simulink model "qss_example_electric"  (Simulink 9.2)
settings: Solver=VariableStepDiscrete  StartTime=0.0  StopTime=1923  RelTol=1e-3  EnableMultiTasking=on
undefined symbols (not defined in the file or in its folder): g, h, P_aux, r_wheel, rho, speed_m_s, trans_eff
libraries: qss_tb_library_aalto x2
settings Model: Creator=Antti  LastModifiedBy=Jesse
settings DataIOCC: LimitDataPoints=off  SaveOutput=off  SaveTime=off
settings OptimizationCC: BooleanDataType=off  ExpressionDepthLimit=2147483647  InitFltsAndDblsToZero=on
settings DebuggingCC: SaveWithParameterizedLinksMsg=none  SignalResolutionControl=TryResolveAllWithWarning  SolverPrmCheckMsg=warning  MultiTaskDSMMsg=warning  MultiTaskCondExecSysMsg=none
settings GRTTargetCC: TargetFcnLib=ansi_tfl_tmw.mat
settings ConfigComp: CovSFcnEnable=off

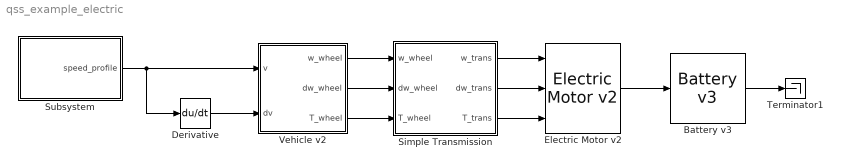
== system qss_example_electric ==
  Battery v3 : qss_tb_library_aalto/Energy Buffer/Battery v3  Tag=battery  init_soc_BT=battery_init_soc  cell_series_BT=192  cell_parallel_BT=25  init_file_BT=battery_file_name
  Derivative : Derivative
  Electric Motor v2 : qss_tb_library_aalto/Energy Converter/Electric Motor v2  scale_EM=3.5  theta_EM=0.5  P_aux=P_aux*1000  over_factor=1.25
  Simple Transmission : Subsystem  Tag=simple transmission  AncestorBlock=qss_tb_library_aalto/Gear System/Simple Transmission  mask(Simple Transmission){gear_ratio=3.5, e_GT=0.98, P_GT0=300, w_wheel_min=1}
      mask prompts: gear_ratio "Gear ratio [-]"; e_GT "Efficiency [-]"; P_GT0 "Idling losses (friction) [W]"; w_wheel_min "Minimum wheel speed beyond which losses are generated [rad/s]"
      mask help:
      | This block simulates a transmission with a fixed gear ratio.
      |
      | Input:
      | =====
      | 	w_wheel	Speed of the wheel [rad/s]
      | 	dw_wheel	Acceleration of the wheel [rad/s^2]
      | 	T_wheel	Torque on the wheel [Nm]
      |
      | Output:
      | ======
      | 	w_trans		Speed of the fly wheel [rad/s]
      | 	dw_trans	Acceleration of the fly wheel [rad/s^2]
      | 	T_trans		Torque on the fly wheel [Nm]
      mask init:
      | init_transmission;
  Subsystem : Subsystem
  Terminator1 : Terminator
  Vehicle v2 : Subsystem  Tag=vehicle  AncestorBlock=qss_tb_library_aalto/Vehicle/Vehicle v2  mask(Vehicle){m_f=1200, mt2m_f=5, A_f=2.0, d_wheel=0.6, cw=0.33, mu=0.01}
      mask prompts: m_f "Total mass of the vehicle [kg]"; mt2m_f "Rotating mass [%]"; A_f "Vehicle cross section [m^2]"; d_wheel "Wheel diameter [m]"; cw "Drag coefficient [-]"; mu "Rolling friction coefficient [-]"
      mask help:
      | This block computes the power required from the vehicle.
      |
      | Input:
      | =====
      | 	v		Speed [m/s]
      | 	dv		Acceleration [m/s^2]
      |
      | Output:
      | ======
      | 	w_wheel	Speed of the wheel [rad/s]
      | 	dw_wheel	Acceleration of the wheel [rad/s^2]
      | 	T_wheel	Torque on the wheel [Nm]
      mask init:
      | init_vehicle_default_v2;
  wires:
  Subsystem/1(speed_profile) -> Vehicle v2/1(v), Derivative/1
  Derivative/1 -> Vehicle v2/2(dv)
  Vehicle v2/1(w_wheel) -> Simple Transmission/1(w_wheel)
  Vehicle v2/2(dw_wheel) -> Simple Transmission/2(dw_wheel)
  Vehicle v2/3(T_wheel) -> Simple Transmission/3(T_wheel)
  Simple Transmission/1(w_trans) -> Electric Motor v2/1
  Simple Transmission/2(dw_trans) -> Electric Motor v2/2
  Simple Transmission/3(T_trans) -> Electric Motor v2/3
  Electric Motor v2/1 -> Battery v3/1
  Battery v3/1 -> Terminator1/1

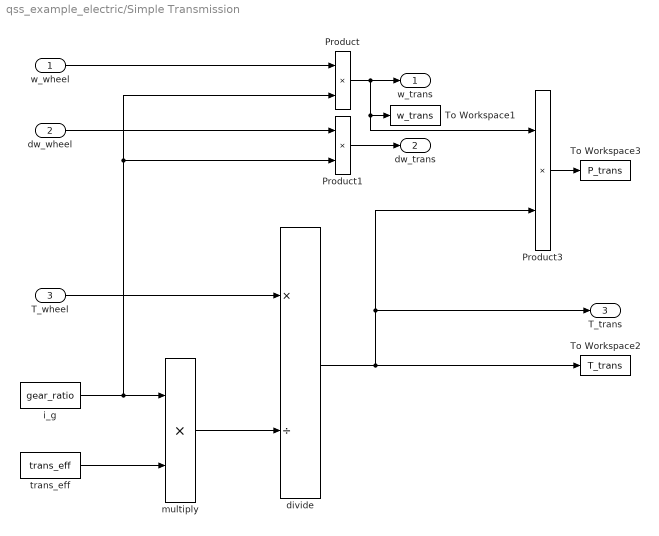
== system qss_example_electric/Simple Transmission ==
  w_wheel : Inport
  dw_wheel : Inport  Port=2
  T_wheel : Inport  Port=3
  Product : Product  SaturateOnIntegerOverflow=on  RndMeth=Zero  InputSameDT=on  OutDataTypeStr=Inherit: Same as first input
  Product1 : Product  SaturateOnIntegerOverflow=on  RndMeth=Zero  InputSameDT=on  OutDataTypeStr=Inherit: Same as first input
  Product3 : Product  SaturateOnIntegerOverflow=on  RndMeth=Zero  InputSameDT=on  OutDataTypeStr=Inherit: Same as first input
  To Workspace1 : ToWorkspace  VariableName=w_trans  SampleTime=-1
  To Workspace2 : ToWorkspace  VariableName=T_trans  SampleTime=-1
  To Workspace3 : ToWorkspace  VariableName=P_trans  SampleTime=-1
  divide : Product  Inputs=*/
  i_g : Constant  Value=gear_ratio
  multiply : Product  Inputs=**
  trans_eff : Constant  Value=trans_eff
  w_trans : Outport  InitialOutput=0
  dw_trans : Outport  Port=2  InitialOutput=0
  T_trans : Outport  Port=3  InitialOutput=0
  wires:
  Product3/1 -> To Workspace3/1
  w_wheel/1 -> Product/1
  dw_wheel/1 -> Product1/1
  Product/1 -> Product3/1, To Workspace1/1, w_trans/1
  Product1/1 -> dw_trans/1
  divide/1 -> Product3/2, T_trans/1, To Workspace2/1
  multiply/1 -> divide/2
  i_g/1 -> Product/2, Product1/2, multiply/1
  trans_eff/1 -> multiply/2
  T_wheel/1 -> divide/1

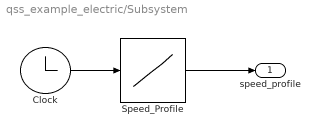
== system qss_example_electric/Subsystem ==
  Clock : Clock
  Speed_Profile : Lookup_n-D  NumberOfTableDimensions=1  BreakpointsSpecification=Even spacing  BreakpointsForDimension1=[0:1923]  Table=speed_m_s  InternalRulePriority=Speed  RndMeth=Simplest  InputSameDT=on
  speed_profile : Outport
  wires:
  Speed_Profile/1 -> speed_profile/1
  Clock/1 -> Speed_Profile/1

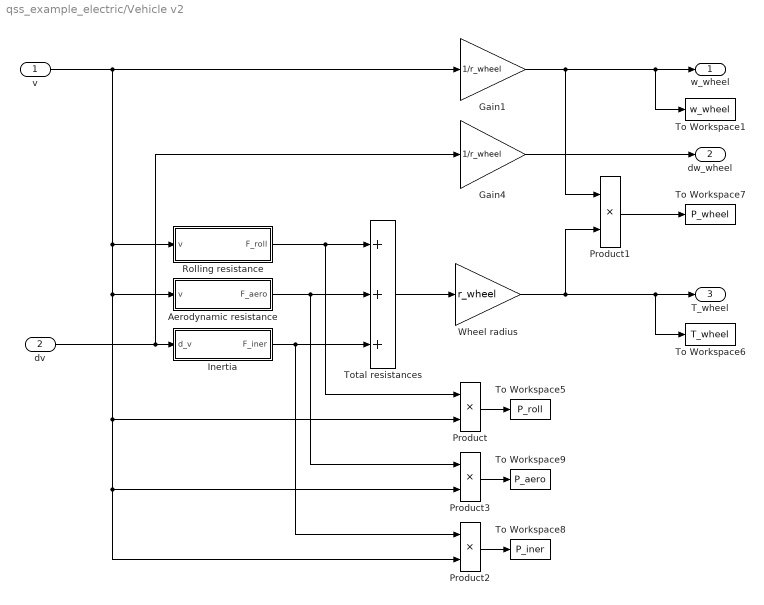
== system qss_example_electric/Vehicle v2 ==
  v : Inport
  dv : Inport  Port=2
  Aerodynamic resistance : Subsystem
  Gain1 : Gain  Gain=1/r_wheel  SaturateOnIntegerOverflow=on  OutDataTypeStr=Inherit: Same as input  ParamDataTypeStr=Inherit: Same as input
  Gain4 : Gain  Gain=1/r_wheel  SaturateOnIntegerOverflow=on  OutDataTypeStr=Inherit: Same as input  ParamDataTypeStr=Inherit: Same as input
  Inertia : Subsystem
  Product{,1..3} (4 alike) : Product  SaturateOnIntegerOverflow=on  RndMeth=Zero  InputSameDT=on  OutDataTypeStr=Inherit: Same as first input
  Rolling resistance : Subsystem
  To Workspace1 : ToWorkspace  VariableName=w_wheel  SampleTime=-1
  To Workspace5 : ToWorkspace  VariableName=P_roll  SampleTime=-1
  To Workspace6 : ToWorkspace  VariableName=T_wheel  SampleTime=-1
  To Workspace7 : ToWorkspace  VariableName=P_wheel  SampleTime=-1
  To Workspace8 : ToWorkspace  VariableName=P_iner  SampleTime=-1
  To Workspace9 : ToWorkspace  VariableName=P_aero  SampleTime=-1
  Total resistances : Sum  Inputs=+++  SaturateOnIntegerOverflow=on  InputSameDT=on  OutDataTypeStr=Inherit: Same as first input
  Wheel radius : Gain  Gain=r_wheel  SaturateOnIntegerOverflow=on  OutDataTypeStr=Inherit: Same as input  ParamDataTypeStr=Inherit: Same as input
  w_wheel : Outport  InitialOutput=0
  dw_wheel : Outport  Port=2  InitialOutput=0
  T_wheel : Outport  Port=3  InitialOutput=0
  wires:
  Gain4/1 -> dw_wheel/1
  Gain1/1 -> Product1/1, w_wheel/1, To Workspace1/1
  Rolling resistance/1(F_roll) -> Total resistances/1, Product/1
  Aerodynamic resistance/1(F_aero) -> Product3/1, Total resistances/2
  Inertia/1(F_iner) -> Total resistances/3, Product2/1
  Total resistances/1 -> Wheel radius/1
  Wheel radius/1 -> Product1/2, T_wheel/1, To Workspace6/1
  v/1 -> Gain1/1, Rolling resistance/1(v), Aerodynamic resistance/1(v), Product/2, Product3/2, Product2/2
  dv/1 -> Inertia/1(d_v), Gain4/1
  Product2/1 -> To Workspace8/1
  Product3/1 -> To Workspace9/1
  Product1/1 -> To Workspace7/1
  Product/1 -> To Workspace5/1

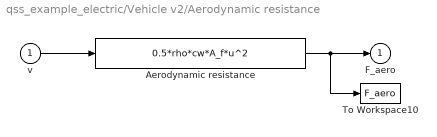
== system qss_example_electric/Vehicle v2/Aerodynamic resistance ==
  v : Inport
  Aerodynamic resistance : Fcn  Expr=0.5*rho*cw*A_f*u^2
  To Workspace10 : ToWorkspace  VariableName=F_aero  SampleTime=-1
  F_aero : Outport  InitialOutput=0
  wires:
  v/1 -> Aerodynamic resistance/1
  Aerodynamic resistance/1 -> F_aero/1, To Workspace10/1

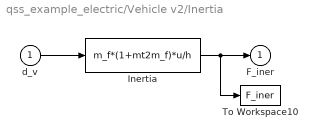
== system qss_example_electric/Vehicle v2/Inertia ==
  d_v : Inport
  Inertia : Fcn  Expr=m_f*(1+mt2m_f)*u/h
  To Workspace10 : ToWorkspace  VariableName=F_iner  SampleTime=-1
  F_iner : Outport  InitialOutput=0
  wires:
  Inertia/1 -> F_iner/1, To Workspace10/1
  d_v/1 -> Inertia/1

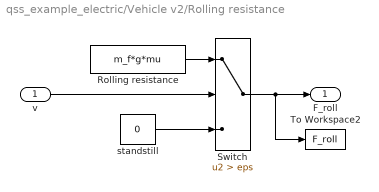
== system qss_example_electric/Vehicle v2/Rolling resistance ==
  v : Inport
  Rolling resistance : Constant  Value=m_f*g*mu
  Switch : Switch  Criteria=u2 > Threshold  Threshold=eps
  To Workspace2 : ToWorkspace  VariableName=F_roll  SampleTime=-1
  standstill : Constant  Value=0
  F_roll : Outport
  wires:
  Switch/1 -> To Workspace2/1, F_roll/1
  v/1 -> Switch/2
  standstill/1 -> Switch/3
  Rolling resistance/1 -> Switch/1
